simulink model "mte484part1e"  (R2024a)
settings: Solver=VariableStepAuto  StartTime=0.0  StopTime=10.0  RelTol=1e-3
values from neighbouring files (symbols this model uses):
  A = 1.0    (= 1)    [mte484part1esetup.m]
  freq = 0.25    [mte484part1esetup.m]
  K1 = 1.883    [mte484part1esetup.m]
  Kp = 3.5    [mte484part1esetup.m]
  sat = 0.7    [mte484part1esetup.m]
  tau = 0.0216    [mte484part1esetup.m]
settings Model: Creator=christopherkoo  LastModifiedBy=christopherkoo

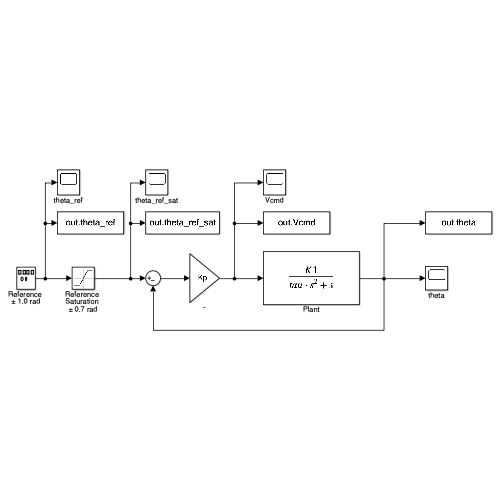
[thumbnail: Simulink's stored preview of the top-level diagram]
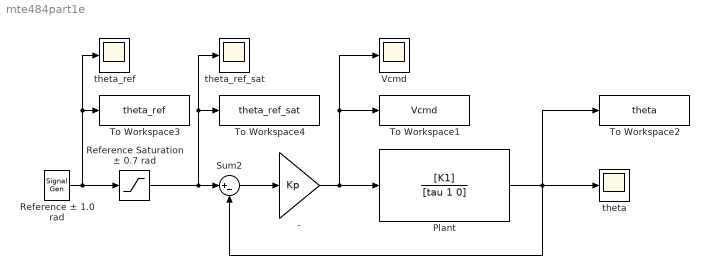
== system mte484part1e ==
  - : Gain  Gain=Kp
  Plant : TransferFcn  Numerator=[K1]  Denominator=[tau 1 0]
  Reference Saturation ± 0.7 rad : Saturate  UpperLimit=sat  LowerLimit=-sat
  Reference ± 1.0 rad : SignalGenerator  WaveForm=square  Amplitude=A  Frequency=freq
  Sum2 : Sum  Inputs=|+-
  To Workspace1 : ToWorkspace  VariableName=Vcmd  SaveFormat=Timeseries  SampleTime=-1
  To Workspace2 : ToWorkspace  VariableName=theta  SaveFormat=Timeseries  SampleTime=-1
  To Workspace3 : ToWorkspace  VariableName=theta_ref  SaveFormat=Timeseries  SampleTime=-1
  To Workspace4 : ToWorkspace  VariableName=theta_ref_sat  SaveFormat=Timeseries  SampleTime=-1
  Vcmd : Scope
  theta : Scope
  theta_ref : Scope
  theta_ref_sat : Scope
  wires:
  Sum2/1 -> -/1
  Plant/1 -> To Workspace2/1, theta/1, Sum2/2
  -/1 -> Plant/1, Vcmd/1, To Workspace1/1
  Reference Saturation ± 0.7 rad/1 -> theta_ref_sat/1, To Workspace4/1, Sum2/1
  Reference ± 1.0 rad/1 -> Reference Saturation ± 0.7 rad/1, theta_ref/1, To Workspace3/1
